simulink model "EnvT_DD"  (R2016b)
settings: configuration reference "CodeGenConfigSet" (kept outside this file)
values from neighbouring files (symbols this model uses):
  EnvT_tiMaxDefDeb_C = Calibration.Parameter    [init_EnvT_DD.m]
  EnvT_tiMaxOKDeb_C = Calibration.Parameter    [init_EnvT_DD.m]
  EnvT_tiMinDefDeb_C = Calibration.Parameter    [init_EnvT_DD.m]
  EnvT_tiMinOKDeb_C = Calibration.Parameter    [init_EnvT_DD.m]
  EnvT_tiPhysRngHiDefDeb_C = Calibration.Parameter    [init_EnvT_DD.m]
  EnvT_tiPhysRngHiOKDeb_C = Calibration.Parameter    [init_EnvT_DD.m]
  EnvT_tiPhysRngLoDefDeb_C = Calibration.Parameter    [init_EnvT_DD.m]
  EnvT_tiPhysRngLoOKDeb_C = Calibration.Parameter    [init_EnvT_DD.m]
  EnvT_tPhysRngMax_C = Calibration.Parameter    [init_EnvT_DD.m]
  EnvT_tPhysRngMin_C = Calibration.Parameter    [init_EnvT_DD.m]
  EnvT_tTransf_CUR = Calibration.Parameter    [init_EnvT_DD.m]
  EnvT_tTransf_CURX = Calibration.Parameter    [init_EnvT_DD.m]
  EnvT_uSRCMax_C = Calibration.Parameter    [init_EnvT_DD.m]
  EnvT_uSRCMin_C = Calibration.Parameter    [init_EnvT_DD.m]
undefined symbols (not defined in the file or in its folder): EnvT_DD_DT
libraries: CXLib x12
settings Model: Creator=lenovo  LastModifiedBy=wangrui
settings ConfigSetRef: SourceLocation=Base Workspace

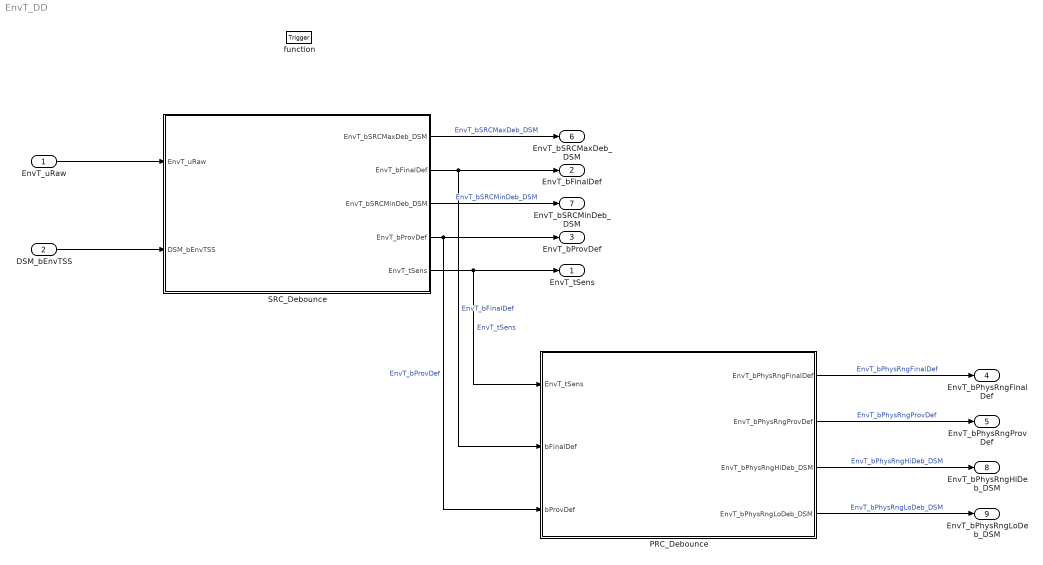
== system EnvT_DD ==
  EnvT_uRaw : Inport  Tag=mv  Description=Sensor signal raw voltage  OutMin=0  OutMax=5000  OutDataTypeStr=Ad_mv
  DSM_bEnvTSS : Inport  Description=state of FId_EnvTSS  Port=2  OutMin=0  OutMax=1  OutDataTypeStr=boolean
  function : TriggerPort  TriggerType=function-call  VariantControl=Variant
  PRC_Debounce : Subsystem
  SRC_Debounce : Subsystem
  EnvT_tSens : Outport  Tag=deg  Description=Raw physical value  OutMin=-200  OutMax=200  OutDataTypeStr=Temp_deg
  EnvT_bFinalDef : Outport  Description=Environment temperature sensor finally defect flag  Port=2  OutMin=0  OutMax=1  OutDataTypeStr=boolean
  EnvT_bProvDef : Outport  Description=Environment temperature sensor temporary defect flag  Port=3  OutMin=0  OutMax=1  OutDataTypeStr=boolean
  EnvT_bPhysRngFinalDef : Outport  Description=Environment temperature sensor physical range finally defect  Port=4  OutMin=0  OutMax=1  OutDataTypeStr=boolean
  EnvT_bPhysRngProvDef : Outport  Description=Environment temperature sensor physical range temporary defect  Port=5  OutMin=0  OutMax=1  OutDataTypeStr=boolean
  EnvT_bSRCMaxDeb_DSM : Outport  Description=SRC-Max error of Environment temperature sensor  Port=6  OutMin=0  OutMax=1  OutDataTypeStr=boolean
  EnvT_bSRCMinDeb_DSM : Outport  Description=SRC-Min error of Environment temperature sensor  Port=7  OutMin=0  OutMax=1  OutDataTypeStr=boolean
  EnvT_bPhysRngHiDeb_DSM : Outport  Description=Physical-High of Environment temperature sensor  Port=8  OutMin=0  OutMax=1  OutDataTypeStr=boolean
  EnvT_bPhysRngLoDeb_DSM : Outport  Description=Physical-Low of Environment temperature sensor  Port=9  OutMin=0  OutMax=1  OutDataTypeStr=boolean
  wires:
  SRC_Debounce/5(EnvT_tSens) -> PRC_Debounce/1(EnvT_tSens), EnvT_tSens/1  "EnvT_tSens"
  EnvT_uRaw/1 -> SRC_Debounce/1(EnvT_uRaw)
  DSM_bEnvTSS/1 -> SRC_Debounce/2(DSM_bEnvTSS)
  SRC_Debounce/1(EnvT_bSRCMaxDeb_DSM) -> EnvT_bSRCMaxDeb_DSM/1  "EnvT_bSRCMaxDeb_DSM"
  SRC_Debounce/2(EnvT_bFinalDef) -> PRC_Debounce/2(bFinalDef), EnvT_bFinalDef/1  "EnvT_bFinalDef"
  SRC_Debounce/3(EnvT_bSRCMinDeb_DSM) -> EnvT_bSRCMinDeb_DSM/1  "EnvT_bSRCMinDeb_DSM"
  SRC_Debounce/4(EnvT_bProvDef) -> PRC_Debounce/3(bProvDef), EnvT_bProvDef/1  "EnvT_bProvDef"
  PRC_Debounce/1(EnvT_bPhysRngFinalDef) -> EnvT_bPhysRngFinalDef/1  "EnvT_bPhysRngFinalDef"
  PRC_Debounce/2(EnvT_bPhysRngProvDef) -> EnvT_bPhysRngProvDef/1  "EnvT_bPhysRngProvDef"
  PRC_Debounce/3(EnvT_bPhysRngHiDeb_DSM) -> EnvT_bPhysRngHiDeb_DSM/1  "EnvT_bPhysRngHiDeb_DSM"
  PRC_Debounce/4(EnvT_bPhysRngLoDeb_DSM) -> EnvT_bPhysRngLoDeb_DSM/1  "EnvT_bPhysRngLoDeb_DSM"

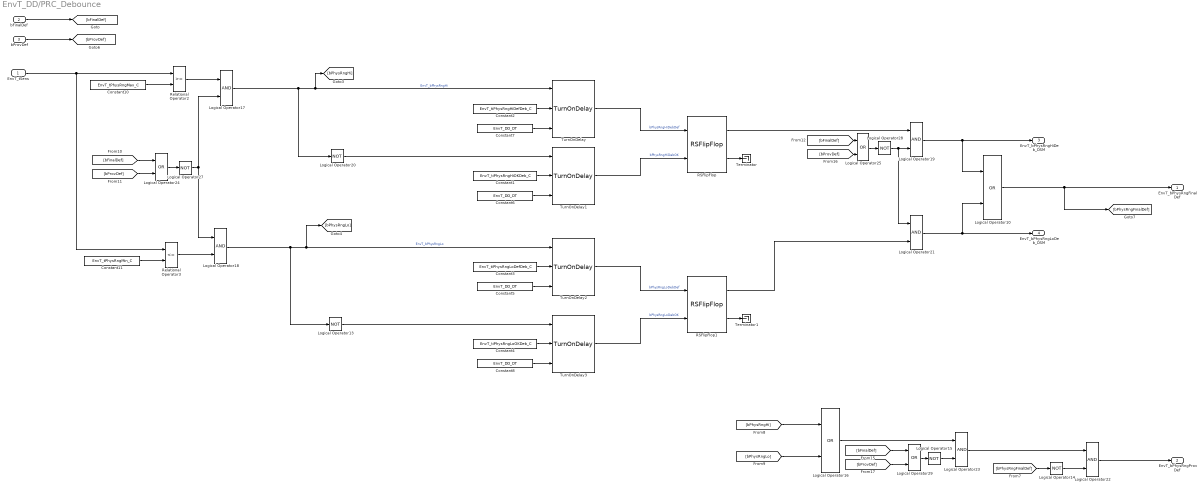
== system EnvT_DD/PRC_Debounce ==
  EnvT_tSens : Inport
  bFinalDef : Inport  Port=2
  bProvDef : Inport  Port=3
  Constant1 : Constant  Value=EnvT_tiPhysRngHiOKDeb_C
  Constant10 : Constant  Value=EnvT_tPhysRngMax_C
  Constant11 : Constant  Value=EnvT_tPhysRngMin_C
  Constant2 : Constant  Value=EnvT_tiPhysRngHiDefDeb_C
  Constant3 : Constant  Value=EnvT_tiPhysRngLoDefDeb_C
  Constant4 : Constant  Value=EnvT_tiPhysRngLoOKDeb_C
  Constant{5..8} (4 alike) : Constant  Value=EnvT_DD_DT  OutDataTypeStr=Inherit: Inherit via back propagation
  Logical Operator10 : Logic  Operator=OR  AllPortsSameDT=off  OutDataTypeStr=boolean
  Logical Operator{13..15,20,27..28} (6 alike) : Logic  Operator=NOT  AllPortsSameDT=off  OutDataTypeStr=boolean
  Logical Operator16 : Logic  Operator=OR  AllPortsSameDT=off  OutDataTypeStr=boolean
  Logical Operator{17..19,21..23} (6 alike) : Logic  AllPortsSameDT=off  OutDataTypeStr=boolean
  Logical Operator24 : Logic  RequirementInfo={} %GIDa_713e3dc0_6f9e_4c44_952d_c96fe7e298be  Operator=OR  OutDataTypeStr=boolean
  Logical Operator25 : Logic  RequirementInfo={} %GIDa_4bfcca31_eded_4688_810b_675582dfc775  Operator=OR  OutDataTypeStr=boolean
  Logical Operator29 : Logic  RequirementInfo={} %GIDa_3144a257_c32e_41b2_9776_388e25425579  Operator=OR  OutDataTypeStr=boolean
  RSFlipFlop : CXLib/RSFlipFlop
  RSFlipFlop1 : CXLib/RSFlipFlop
  Relational Operator2 : RelationalOperator  OutDataTypeStr=boolean  RndMeth=Nearest  InputSameDT=on
  Relational Operator3 : RelationalOperator  Operator=<=  OutDataTypeStr=boolean  RndMeth=Nearest  InputSameDT=on
  Terminator : Terminator
  Terminator1 : Terminator
  TurnOnDelay{,1..3} (4 alike) : CXLib/TurnOnDelay
  EnvT_bPhysRngFinalDef : Outport  OutMin=0  OutMax=1  OutDataTypeStr=boolean
  EnvT_bPhysRngProvDef : Outport  Port=2  OutMin=0  OutMax=1  OutDataTypeStr=boolean
  EnvT_bPhysRngHiDeb_DSM : Outport  Port=3  OutMin=0  OutMax=1  OutDataTypeStr=boolean
  EnvT_bPhysRngLoDeb_DSM : Outport  Port=4  OutMin=0  OutMax=1  OutDataTypeStr=boolean
  wires:
  Logical Operator15/1 -> Logical Operator23/2
  Logical Operator10/1 -> EnvT_bPhysRngFinalDef/1, [bPhysRngFinalDef]
  Logical Operator16/1 -> Logical Operator23/1
  Logical Operator24/1 -> Logical Operator27/1
  Logical Operator25/1 -> Logical Operator28/1
  RSFlipFlop/1 -> Logical Operator19/1
  [bProvDef] -> Logical Operator24/2
  [bFinalDef] -> Logical Operator24/1
  [bProvDef] -> Logical Operator29/2
  Logical Operator27/1 -> Logical Operator17/2, Logical Operator18/1
  [bProvDef] -> Logical Operator25/2
  [bPhysRngHi] -> Logical Operator16/1
  [bPhysRngLo] -> Logical Operator16/2
  Logical Operator19/1 -> EnvT_bPhysRngHiDeb_DSM/1, Logical Operator10/1
  Logical Operator18/1 -> Logical Operator13/1, [bPhysRngLo], TurnOnDelay2/1  "EnvT_bPhysRngLo"
  Logical Operator21/1 -> EnvT_bPhysRngLoDeb_DSM/1, Logical Operator10/2
  [bFinalDef] -> Logical Operator25/1
  Constant11/1 -> Relational Operator3/2
  Logical Operator29/1 -> Logical Operator15/1
  Logical Operator17/1 -> Logical Operator20/1, [bPhysRngHi], TurnOnDelay/1  "EnvT_bPhysRngHi"
  Logical Operator14/1 -> Logical Operator22/2
  Logical Operator23/1 -> Logical Operator22/1
  Logical Operator22/1 -> EnvT_bPhysRngProvDef/1
  Constant10/1 -> Relational Operator2/2
  Logical Operator28/1 -> Logical Operator19/2, Logical Operator21/1
  RSFlipFlop1/1 -> Logical Operator21/2
  Relational Operator2/1 -> Logical Operator17/1
  [bPhysRngFinalDef] -> Logical Operator14/1
  Relational Operator3/1 -> Logical Operator18/2
  [bFinalDef] -> Logical Operator29/1
  EnvT_tSens/1 -> Relational Operator3/1, Relational Operator2/1
  bFinalDef/1 -> [bFinalDef]
  bProvDef/1 -> [bProvDef]
  Constant8/1 -> TurnOnDelay3/3
  Constant5/1 -> TurnOnDelay2/3
  Constant6/1 -> TurnOnDelay1/3
  Constant7/1 -> TurnOnDelay/3
  TurnOnDelay1/1 -> RSFlipFlop/2  "bPhysRngHiDebOK"
  Constant3/1 -> TurnOnDelay2/2
  Constant1/1 -> TurnOnDelay1/2
  Constant2/1 -> TurnOnDelay/2
  TurnOnDelay/1 -> RSFlipFlop/1  "bPhysRngHiDebDef"
  Logical Operator20/1 -> TurnOnDelay1/1
  TurnOnDelay2/1 -> RSFlipFlop1/1  "bPhysRngLoDebDef"
  Logical Operator13/1 -> TurnOnDelay3/1
  TurnOnDelay3/1 -> RSFlipFlop1/2  "bPhysRngLoDebOK"
  Constant4/1 -> TurnOnDelay3/2
  RSFlipFlop/2 -> Terminator/1
  RSFlipFlop1/2 -> Terminator1/1

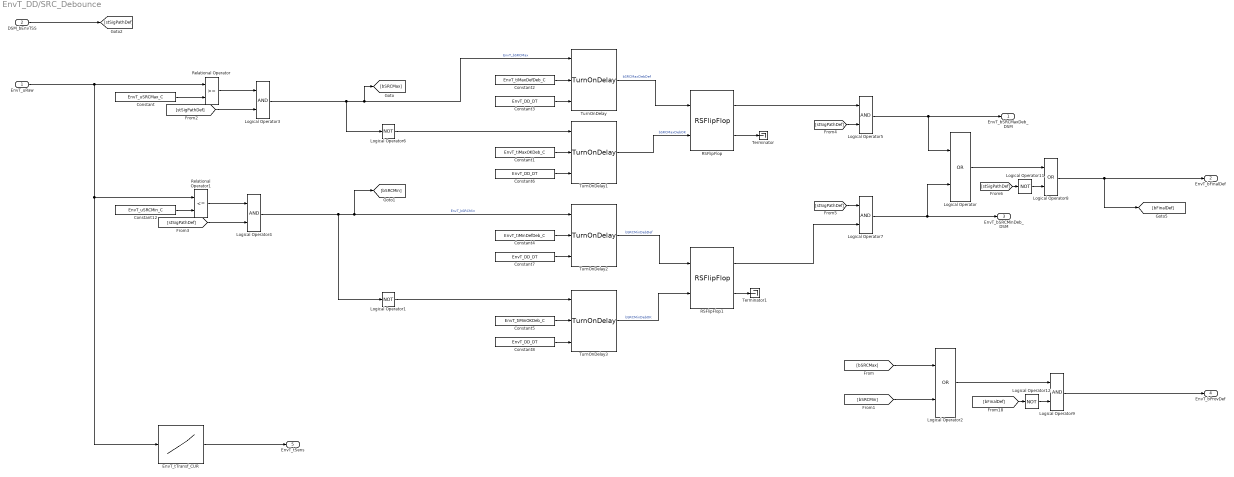
== system EnvT_DD/SRC_Debounce ==
  EnvT_uRaw : Inport  Tag=mv  Description=Sensor signal raw voltage  OutMin=0  OutMax=5000  OutDataTypeStr=Ad_mv
  DSM_bEnvTSS : Inport  Description=state of FId_EnvTSS  Port=2  OutMin=0  OutMax=1  OutDataTypeStr=boolean
  Constant : Constant  Value=EnvT_uSRCMax_C
  Constant1 : Constant  Value=EnvT_tiMaxOKDeb_C
  Constant12 : Constant  Value=EnvT_uSRCMin_C
  Constant2 : Constant  Value=EnvT_tiMaxDefDeb_C
  Constant{3,6..8} (4 alike) : Constant  Value=EnvT_DD_DT  OutDataTypeStr=Inherit: Inherit via back propagation
  Constant4 : Constant  Value=EnvT_tiMinDefDeb_C
  Constant5 : Constant  Value=EnvT_tiMinOKDeb_C
  EnvT_tTransf_CUR : Lookup_n-D  NumberOfTableDimensions=1  BreakpointsForDimension1=EnvT_tTransf_CURX  IndexSearchMethod=Linear search  BeginIndexSearchUsingPreviousIndexResult=on  UseOneInputPortForAllInputData=on  Table=EnvT_tTransf_CUR  ExtrapMethod=Clip  UseLastTableValue=on  InternalRulePriority=Speed  OutDataTypeStr=Inherit: Inherit via back propagation  SaturateOnIntegerOverflow=on
  Logical Operator : Logic  Operator=OR  AllPortsSameDT=off  OutDataTypeStr=boolean
  Logical Operator{1,6,11..12} (4 alike) : Logic  Operator=NOT  AllPortsSameDT=off  OutDataTypeStr=boolean
  Logical Operator2 : Logic  Operator=OR  AllPortsSameDT=off  OutDataTypeStr=boolean
  Logical Operator{3..5,7,9} (5 alike) : Logic  AllPortsSameDT=off  OutDataTypeStr=boolean
  Logical Operator8 : Logic  Operator=OR  AllPortsSameDT=off  OutDataTypeStr=boolean
  RSFlipFlop : CXLib/RSFlipFlop
  RSFlipFlop1 : CXLib/RSFlipFlop
  Relational Operator : RelationalOperator  OutDataTypeStr=boolean  RndMeth=Nearest  InputSameDT=on
  Relational Operator1 : RelationalOperator  Operator=<=  OutDataTypeStr=boolean  RndMeth=Nearest  InputSameDT=on
  Terminator : Terminator
  Terminator1 : Terminator
  TurnOnDelay{,1..3} (4 alike) : CXLib/TurnOnDelay
  EnvT_bSRCMaxDeb_DSM : Outport  OutMin=0  OutMax=1  OutDataTypeStr=boolean
  EnvT_bFinalDef : Outport  Port=2  OutMin=0  OutMax=1  OutDataTypeStr=boolean
  EnvT_bSRCMinDeb_DSM : Outport  Port=3  OutMin=0  OutMax=1  OutDataTypeStr=boolean
  EnvT_bProvDef : Outport  Port=4  OutMin=0  OutMax=1  OutDataTypeStr=boolean
  EnvT_tSens : Outport  Tag=deg  Description=Raw physical value  Port=5  OutMin=-200  OutMax=200  OutDataTypeStr=Temp_deg
  wires:
  Constant/1 -> Relational Operator/2
  Constant12/1 -> Relational Operator1/2
  Logical Operator4/1 -> TurnOnDelay2/1, [bSRCMin], Logical Operator1/1  "EnvT_bSRCMin"
  Logical Operator3/1 -> TurnOnDelay/1, [bSRCMax], Logical Operator6/1  "EnvT_bSRCMax"
  [stSigPathDef] -> Logical Operator11/1
  Logical Operator/1 -> Logical Operator8/1
  [stSigPathDef] -> Logical Operator5/2
  [stSigPathDef] -> Logical Operator7/1
  [stSigPathDef] -> Logical Operator4/2
  Relational Operator/1 -> Logical Operator3/1
  Relational Operator1/1 -> Logical Operator4/1
  [stSigPathDef] -> Logical Operator3/2
  [bSRCMin] -> Logical Operator2/2
  DSM_bEnvTSS/1 -> [stSigPathDef]
  Logical Operator5/1 -> EnvT_bSRCMaxDeb_DSM/1, Logical Operator/1
  [bSRCMax] -> Logical Operator2/1
  Logical Operator7/1 -> EnvT_bSRCMinDeb_DSM/1, Logical Operator/2
  EnvT_tTransf_CUR/1 -> EnvT_tSens/1
  RSFlipFlop1/1 -> Logical Operator7/2
  RSFlipFlop/1 -> Logical Operator5/1
  EnvT_uRaw/1 -> Relational Operator/1, Relational Operator1/1, EnvT_tTransf_CUR/1
  Logical Operator12/1 -> Logical Operator9/2
  Logical Operator11/1 -> Logical Operator8/2
  Logical Operator9/1 -> EnvT_bProvDef/1
  Logical Operator8/1 -> EnvT_bFinalDef/1, [bFinalDef]
  [bFinalDef] -> Logical Operator12/1
  Logical Operator2/1 -> Logical Operator9/1
  Constant8/1 -> TurnOnDelay3/3
  Constant7/1 -> TurnOnDelay2/3
  Constant3/1 -> TurnOnDelay/3
  Constant6/1 -> TurnOnDelay1/3
  RSFlipFlop1/2 -> Terminator1/1
  RSFlipFlop/2 -> Terminator/1
  Constant5/1 -> TurnOnDelay3/2
  TurnOnDelay3/1 -> RSFlipFlop1/2  "bSRCMinDebOK"
  Logical Operator1/1 -> TurnOnDelay3/1
  TurnOnDelay2/1 -> RSFlipFlop1/1  "bSRCMinDebDef"
  Logical Operator6/1 -> TurnOnDelay1/1
  TurnOnDelay/1 -> RSFlipFlop/1  "bSRCMaxDebDef"
  Constant2/1 -> TurnOnDelay/2
  Constant1/1 -> TurnOnDelay1/2
  Constant4/1 -> TurnOnDelay2/2
  TurnOnDelay1/1 -> RSFlipFlop/2  "bSRCMaxDebOK"
